simulink model "LoadFlow58BusNetwork_2023"  (R2023b)
settings: Solver=FixedStepDiscrete  StartTime=0.0  StopTime=4.5  FixedStep=75e-6  RelTol=1e-3  EnableMultiTasking=on
undefined symbols (not defined in the file): D1, D11, Delta
libraries: spsSeriesRLCBranchLib x41, spsLoadFlowBusLib x29, spsDistributedParametersLineLib x19, spsThreePhaseSeriesRLCLoadLib x15, spsThreePhaseTransformerTwoWindingsLib x13, spsThreePhaseParallelRLCLoadLib x11, spsThreePhaseVIMeasurementLib x11, spsSynchronousMachinepuStandardLib x7, spsExcitationSystemLib x7, spsHydraulicTurbineandGovernorLib x7, spsGenericPowerSystemStabilizerLib x7, spsMultiBandPowerSystemStabilizerLib x7
(part 2 of 5)

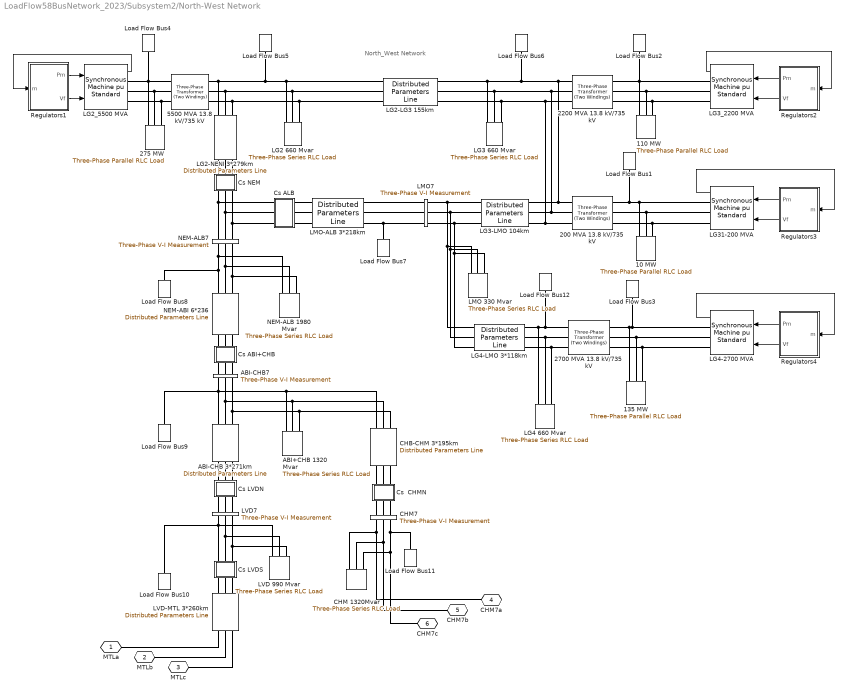
== system LoadFlow58BusNetwork_2023/Subsystem2/North-West Network ==
  note: North_West Network
  10 MW : spsThreePhaseParallelRLCLoadLib/Three-Phase Parallel RLC Load  LConnTagsString=A|B|C  Configuration=Y (grounded)  NominalVoltage=(13800)*1  Vabc=[1e3 1e3 1e3]  Vabcp=[1e3 1e3 1e3]  NominalFrequency=60  UnbalancedPower=off  ActivePower=10000000  InductivePower=0  CapacitivePower=0  Pabc=[10e3 9e3 11e3]  QLabc=[100 90 110]  QCabc=[100 90 110]  Pabcp=[10e3 9e3 11e3]  QLabcp=[100 90 110]  QCabcp=[100 90 110]  Measurements=None  LoadType=constant PQ
  110 MW : spsThreePhaseParallelRLCLoadLib/Three-Phase Parallel RLC Load  LConnTagsString=A|B|C  Configuration=Y (grounded)  NominalVoltage=(13800)*1  Vabc=[1e3 1e3 1e3]  Vabcp=[1e3 1e3 1e3]  NominalFrequency=60  UnbalancedPower=off  ActivePower=110000000  InductivePower=0  CapacitivePower=0  Pabc=[10e3 9e3 11e3]  QLabc=[100 90 110]  QCabc=[100 90 110]  Pabcp=[10e3 9e3 11e3]  QLabcp=[100 90 110]  QCabcp=[100 90 110]  Measurements=None  LoadType=constant PQ
  135 MW : spsThreePhaseParallelRLCLoadLib/Three-Phase Parallel RLC Load  LConnTagsString=A|B|C  Configuration=Y (grounded)  NominalVoltage=(13800)*1  Vabc=[1e3 1e3 1e3]  Vabcp=[1e3 1e3 1e3]  NominalFrequency=60  UnbalancedPower=off  ActivePower=135000000  InductivePower=0  CapacitivePower=0  Pabc=[10e3 9e3 11e3]  QLabc=[100 90 110]  QCabc=[100 90 110]  Pabcp=[10e3 9e3 11e3]  QLabcp=[100 90 110]  QCabcp=[100 90 110]  Measurements=None  LoadType=constant PQ
  200 MVA 13.8 kV/735 kV : spsThreePhaseTransformerTwoWindingsLib/Three-Phase Transformer (Two Windings)  Winding1Connection=Delta (D1)  Winding2Connection=Yg  CoreType=Three single-phase transformers  SetSaturation=off  Hysteresis=off  DataFile='basic_model'  SetInitialFlux=off  Measurements=None  UNITS=pu  NominalPower=[ 200e6 60 ]  Winding1="[ 13.8e3 0.002  0.0]"  Winding2=[ 735e3 0.002 0.12]  Rm=500  Lm=500  L0=0.5  Saturation="[ 0,0  ;  0.005,1.2  ;  1.0,1.4 ]"  InitialFluxes=[ 0.8 , -0.8 , 0.7 ]  BreakLoop=off  DiscreteSolver=Trapezoidal iterative  DataType=off  TransfoNumber=0
  2200 MVA 13.8 kV/735 kV : spsThreePhaseTransformerTwoWindingsLib/Three-Phase Transformer (Two Windings)  Winding1Connection=Delta (D1)  Winding2Connection=Yg  CoreType=Three single-phase transformers  SetSaturation=off  Hysteresis=off  DataFile='basic_model'  SetInitialFlux=off  Measurements=None  UNITS=pu  NominalPower=[ 2200e6 60 ]  Winding1="[ 13.8e3 0.002  0.0]"  Winding2=[ 735e3 0.002 0.12]  Rm=500  Lm=500  L0=0.5  Saturation="[ 0,0  ;  0.005,1.2  ;  1.0,1.4 ]"  InitialFluxes=[ 0.8 , -0.8 , 0.7 ]  BreakLoop=off  DiscreteSolver=Trapezoidal iterative  DataType=off  TransfoNumber=0
  2700 MVA 13.8 kV/735 kV : spsThreePhaseTransformerTwoWindingsLib/Three-Phase Transformer (Two Windings)  Winding1Connection=Delta (D1)  Winding2Connection=Yg  CoreType=Three single-phase transformers  SetSaturation=off  Hysteresis=off  DataFile='basic_model'  SetInitialFlux=off  Measurements=None  UNITS=pu  NominalPower=[ 2700e6 60 ]  Winding1="[ 13.8e3 0.002  0.0]"  Winding2=[ 735e3 0.002 0.12]  Rm=500  Lm=500  L0=0.5  Saturation="[ 0,0  ;  0.005,1.2  ;  1.0,1.4 ]"  InitialFluxes=[ 0.8 , -0.8 , 0.7 ]  BreakLoop=off  DiscreteSolver=Trapezoidal iterative  DataType=off  TransfoNumber=0
  275 MW : spsThreePhaseParallelRLCLoadLib/Three-Phase Parallel RLC Load  LConnTagsString=A|B|C  Configuration=Y (grounded)  NominalVoltage=(13800)*1  Vabc=[1e3 1e3 1e3]  Vabcp=[1e3 1e3 1e3]  NominalFrequency=60  UnbalancedPower=off  ActivePower=275000000  InductivePower=0  CapacitivePower=0  Pabc=[10e3 9e3 11e3]  QLabc=[100 90 110]  QCabc=[100 90 110]  Pabcp=[10e3 9e3 11e3]  QLabcp=[100 90 110]  QCabcp=[100 90 110]  Measurements=None  LoadType=constant PQ
  5500 MVA 13.8 kV/735 kV : spsThreePhaseTransformerTwoWindingsLib/Three-Phase Transformer (Two Windings)  Winding1Connection=Delta (D1)  Winding2Connection=Yg  CoreType=Three single-phase transformers  SetSaturation=off  Hysteresis=off  DataFile='basic_model'  SetInitialFlux=off  Measurements=None  UNITS=pu  NominalPower=[ 5500e6 60 ]  Winding1="[ 13.8e3 0.002  0.0]"  Winding2=[ 735e3 0.002 0.12]  Rm=500  Lm=500  L0=0.5  Saturation="[ 0,0  ;  0.005,1.2  ;  1.0,1.4 ]"  InitialFluxes=[ 0.8 , -0.8 , 0.7 ]  BreakLoop=off  DiscreteSolver=Trapezoidal iterative  DataType=off  TransfoNumber=0
  ABI+CHB 1320 Mvar : spsThreePhaseSeriesRLCLoadLib/Three-Phase Series RLC Load  LConnTagsString=A|B|C  Configuration=Y (grounded)  NominalVoltage=735e3  Vabc=[1e3 1e3 1e3]  Vabcp=[1e3 1e3 1e3]  NominalFrequency=60  UnbalancedPower=off  ActivePower=4400000  InductivePower=1320e6  CapacitivePower=0  Pabc=[10e3 9e3 11e3]  QLabc=[100 90 110]  QCabc=[100 90 110]  Pabcp=[10e3 9e3 11e3]  QLabcp=[100 90 110]  QCabcp=[100 90 110]  Measurements=None  LoadType=constant Z
  ABI-CHB 3*271km : spsDistributedParametersLineLib/Distributed Parameters Line  Phases=3  Length=271  Frequency=60  Resistance="[0.01273  0.3864]/3"  Inductance="[0.9337e-3  4.1264e-3]/3"  Capacitance=[12.74e-9 7.751e-9]*3  x1=[-0.001575 2.66910784944011e-08 -34814.2579740562 -747194.944177999;-0.0015 2.68155154258362e-08 -13676.7298713595 -747880.497252668;-0.001425 2.69185164445309e-08 7471.73119993543 -747968.206100789;-0.00135 2.6999999213047e-08 28614.2194836304 -747458.00060925;-0.001275 2.70598985953061e-08 49733.8339980823 -746350.288628515;-0.0012 2.70981667086584e-08 70813.6920465894 -744645.955646593;-0.001125 2.71147729621596e-08 91836.9427131602 -742346.364081192;-0.00105 2.71097040810249e-08 112786.780332879 -739453.352190625;-0.000975 2.70829641172401e-08 133646.457926094 -735969.232604332;-0.0009 2.70345744463233e-08 154399.300585704 -731896.790474202;-0.000825 2.69645737502369e-08 175028.718806813 -727239.281248164;-0.00075 2.68730179864664e-08 195518.221748137 -722000.428067829;-0.000675 2.67599803432885e-08 215851.430414525 -716184.418792275;-0.0006 2.66255511812656e-08 236012.090750078 -709795.902650327;-0.000525 2.6469837961013e-08 255984.08663139 -702839.986524042;-0.00045 2.62929651572965e-08 275751.452750538 -695322.230866342;-0.000375 2.60950741595291e-08 295298.387377495 -687248.645256074;-0.0003 2.58763231587465e-08 314609.2649918 -678625.683594045;-0.000225 2.56368870211519e-08 333668.648773354 -669460.238943873;-0.00015 2.53769571483301e-08 352461.302942379 -659759.638021774;-7.5e-05 2.50967413242444e-08 370972.204938671 -649531.635339701]  x2=[-0.001575 6.08393924870088e-08 -284619.34107611 -691578.758256664;-0.0015 6.10523834949351e-08 -264954.255311304 -699348.683850969;-0.001425 6.12165701616285e-08 -245077.369168738 -706559.560807798;-0.00135 6.13318212387795e-08 -225004.571927068 -713205.62486244;-0.001275 6.13980445964407e-08 -204751.909473285 -719281.56325298;-0.0012 6.1415187296673e-08 -184335.571475878 -724782.518967232;-0.001125 6.13832356358642e-08 -163771.878443063 -729704.094625366;-0.00105 6.13022151556831e-08 -143077.268676413 -734042.355995104;-0.000975 6.11721906226619e-08 -122268.28513034 -737793.835136684;-0.0009 6.09932659764228e-08 -101361.5621879 -740955.53317508;-0.000825 6.07655842465905e-08 -80373.812363532 -743524.922697255;-0.00075 6.0489327438456e-08 -59321.8129433208 -745499.94977254;-0.000675 6.0164716387485e-08 -38222.3925734968 -746879.035594507;-0.0006 5.97920105827849e-08 -17092.4178078718 -747661.077743053;-0.000525 5.93715079596733e-08 4051.22037502602 -747845.45106565;-0.00045 5.89035446615133e-08 25191.6200743418 -747432.008177083;-0.000375 5.83884947710054e-08 46311.8819780149 -746421.079577273;-0.0003 5.78267700111514e-08 67395.1228718303 -744813.473387074;-0.000225 5.72188194161298e-08 88424.489135602 -742610.474702278;-0.00015 5.65651289723442e-08 109383.170215699 -739813.844566326;-7.5e-05 5.58662212299336e-08 130254.412063144 -736425.81856256]  x3=[-0.001575 1.19957394580366e-10 -354.9640306607 -109.750554354856;-0.0015 1.27832366196785e-10 -351.719210477087 -119.74113183903;-0.001425 1.35605150575568e-10 -348.193231338104 -129.635990094512;-0.00135 1.43269534271808e-10 -344.388911857524 -139.427219323009;-0.001275 1.50819390494449e-10 -340.309293150132 -149.106992565688;-0.0012 1.58248684003943e-10 -335.957636400702 -158.667571959923;-0.001125 1.65551475936731e-10 -331.337420257058 -168.101314924829;-0.00105 1.72721928552677e-10 -326.452338049293 -177.40068027062;-0.000975 1.79754309901672e-10 -321.30629483738 -186.558234226925;-0.0009 1.86642998405664e-10 -315.903404289525 -195.566656385225;-0.000825 1.93382487352465e-10 -310.247985393765 -204.41874555068;-0.00075 1.99967389297728e-10 -304.344559005434 -213.107425498655;-0.000675 2.0639244037159e-10 -298.197844233263 -221.625750631338;-0.0006 2.12652504486529e-10 -291.812754666991 -229.966911529955;-0.000525 2.18742577443073e-10 -285.194394449524 -238.124240398106;-0.00045 2.24657790930084e-10 -278.348054196754 -246.091216391906;-0.000375 2.30393416416404e-10 -271.279206768327 -253.861470832645;-0.0003 2.35944868930779e-10 -263.993502892721 -261.42879229781;-0.000225 2.41307710727008e-10 -256.496766650139 -268.787131586407;-0.00015 2.46477654831413e-10 -248.794990816828 -275.930606554595;-7.5e-05 2.51450568469781e-10 -240.89433207455 -282.853506817784]  x4=[-0.001575 1.87301646960915e-10 -5971.27343085188 -15054.8004559029;-0.0015 1.83445794549808e-10 -5543.27939856518 -15217.5948036273;-0.001425 1.79443298377354e-10 -5110.85415354227 -15368.2244389028;-0.00135 1.75297357977751e-10 -4674.34336990772 -15506.5689507035;-0.001275 1.7101128755232e-10 -4234.09598770311 -15632.5177485434;-0.0012 1.6658851332018e-10 -3790.46393394978 -15745.9701508807;-0.001125 1.62032570779382e-10 -3343.80184132369 -15846.8354656009;-0.00105 1.57347101880685e-10 -2894.46676466753 -15935.0330625145;-0.000975 1.52535852116235e-10 -2442.81789556652 -16010.4924378121;-0.0009 1.4760266752548e-10 -1989.21627521616 -16073.1532704238;-0.000825 1.42551491620702e-10 -1534.02450581142 -16122.9654702385;-0.00075 1.37386362234634e-10 -1077.60646068811 -16159.8892181459;-0.000675 1.32111408292677e-10 -620.326993448042 -16183.894997867;-0.0006 1.26730846512303e-10 -162.551646300739 -16194.9636195487;-0.000525 1.21248978032274e-10 295.353642145493 -16193.0862351041;-0.00045 1.15670184974377e-10 753.022829409257 -16178.2643452858;-0.000375 1.09998926940426e-10 1210.09006174483 -16150.5097984855;-0.0003 1.04239737447318e-10 1666.18996660004 -16109.8447812635;-0.000225 9.83972203030162e-11 2120.95794468951 -16056.3018006122;-0.00015 9.24760459263322e-11 2574.03046144974 -15989.9236579711;-7.5e-05 8.64809476134656e-11 3025.04533764307 -15910.7634150119]  x5=0.00153261764655846  V1=ones(3,3)  V2=ones(3,3)  I1=ones(3,3)  I2=ones(3,3)  nHarmo=1  Measurements=None  Decoupling=on  VsMag0=[610743.955114479 610743.501375024 610743.958218046]  VrMag0=[610622.360478008 610622.247686734 610622.21400369]  VsAngle0=[1.35232982185643 -118.647645266058 121.352379141739]  VrAngle0=[-18.3496130787562 -138.349622838578 101.650391206836]  IsMag0=[305.299965909812 305.301188712511 305.286778309358]  IrMag0=[13308.311716937 13308.3164139131 13308.3246262138]  IsAngle0=[-68.7963830006793 171.200626740014 51.2019231191923]  IrAngle0=[-17.6151010152127 -137.615048514483 102.384907722655]
      settings: AttributesFormatString=\n  LibrarySourceBlock=sps_lib/Power Grid Elements/Distributed Parameters Line
  ABI-CHB7 : spsThreePhaseVIMeasurementLib/Three-Phase V-I Measurement  VoltageMeasurement=no  SetLabelV=on  LabelV=Vabc_ABI7  Vpu=on  VpuLL=off  CurrentMeasurement=no  SetLabelI=off  LabelI=A1  Ipu=off  Pbase=100e6  Vbase=500e3  OutputType=Magnitude  PhasorSimulation=off  PSBequivalent=0
  CHB-CHM 3*195km : spsDistributedParametersLineLib/Distributed Parameters Line  Phases=3  Length=195  Frequency=60  Resistance="[0.01273  0.3864]/3"  Inductance="[0.9337e-3  4.1264e-3]/3"  Capacitance=[12.74e-9 7.751e-9]*3  x1=[-0.001125 2.71147729621596e-08 0 0;-0.00105 2.71097040810249e-08 0 0;-0.000975 2.70829641172401e-08 0 0;-0.0009 2.70345744463233e-08 0 0;-0.000825 2.69645737502369e-08 0 0;-0.00075 2.68730179864664e-08 0 0;-0.000675 2.67599803432885e-08 215851.430414525 -716184.418792275;-0.0006 2.66255511812656e-08 236012.090750078 -709795.902650327;-0.000525 2.6469837961013e-08 255984.08663139 -702839.986524042;-0.00045 2.62929651572965e-08 275751.452750538 -695322.230866342;-0.000375 2.60950741595291e-08 295298.387377495 -687248.645256074;-0.0003 2.58763231587465e-08 314609.2649918 -678625.683594045;-0.000225 2.56368870211519e-08 333668.648773354 -669460.238943873;-0.00015 2.53769571483301e-08 352461.302942379 -659759.638021774;-7.5e-05 2.50967413242444e-08 370972.204938671 -649531.635339701]  x2=[-0.001125 1.81716346267298e-08 0 0;-0.00105 1.81182749100996e-08 0 0;-0.000975 1.80504317217251e-08 0 0;-0.0009 1.79681592944132e-08 0 0;-0.000825 1.78715233954833e-08 0 0;-0.00075 1.77606012741946e-08 0 0;-0.000675 1.76354815999936e-08 127559.107191262 -726636.134488437;-0.0006 1.74962643916335e-08 148050.539525883 -722739.535823106;-0.000525 1.73430609372205e-08 168423.622524456 -718265.190231125;-0.00045 1.7175993705252e-08 188662.07025615 -713216.674435898;-0.000375 1.69951962467171e-08 208749.704415509 -707598.024143708;-0.0003 1.68008130883378e-08 228670.467255135 -701413.730817631;-0.000225 1.65929996170367e-08 248408.434422013 -694668.738087127;-0.00015 1.63719219557232e-08 267947.82768719 -687368.437796186;-7.5e-05 1.61377568304971e-08 287273.027558654 -679518.665693159]  x3=[-0.001125 1.00282083292002e-10 0 0;-0.00105 9.83539884232109e-11 0 0;-0.000975 9.63472708809408e-11 0 0;-0.0009 9.42635348044912e-11 0 0;-0.000825 9.21044459005992e-11 0 0;-0.00075 8.98717301118996e-11 0 0;-0.000675 8.75671722372322e-11 771.180648774941 -4323.83757003434;-0.0006 8.5192614504901e-11 893.110598565729 -4300.30718909173;-0.000525 8.27499551000252e-11 1014.32660940907 -4273.33920837907;-0.00045 8.02411466471593e-11 1134.73178308058 -4242.95518568751;-0.000375 7.76681946493944e-11 1254.22986952666 -4209.17940953991;-0.0003 7.50331558851899e-11 1372.72534380541 -4172.03887977492;-0.000225 7.23381367642166e-11 1490.12348244772 -4131.56328596378;-0.00015 6.95852916435246e-11 1606.33043917781 -4087.78498367688;-7.5e-05 6.67768211053835e-11 1721.25331993251 -4040.73896861923]  x4=[-0.001125 6.8922255092171e-11 0 0;-0.00105 7.14623317195361e-11 0 0;-0.000975 7.39452824523348e-11 0 0;-0.0009 7.6369122457742e-11 0 0;-0.000825 7.87319141551432e-11 0 0;-0.00075 8.10317687650074e-11 0 0;-0.000675 8.32668478187486e-11 979.606952616721 -12037.6056406815;-0.0006 8.54353646283689e-11 1319.52443201704 -12005.1005057404;-0.000525 8.75355857147102e-11 1658.38710377581 -11962.9986771393;-0.00045 8.95658321931705e-11 1995.924086258 -11911.3338104356;-0.000375 9.15244811157788e-11 2331.86555756429 -11850.1472057335;-0.0003 9.34099667685547e-11 2665.9429712226 -11779.4877746684;-0.000225 9.52207819231163e-11 2997.88927086002 -11699.4120013084;-0.00015 9.69554790415353e-11 3327.43910368355 -11609.9838970016;-7.5e-05 9.8612671433477e-11 3654.32903259912 -11511.2749492062]  x5=0.0011028060556417  V1=ones(3,3)  V2=ones(3,3)  I1=ones(3,3)  I2=ones(3,3)  nHarmo=1  Measurements=None  Decoupling=on  VsMag0=[610743.955114479 610743.501375024 610743.958218046]  VrMag0=[602368.350238872 602368.356498677 602368.322152189]  VsAngle0=[1.35232982185643 -118.647645266058 121.352379141739]  VrAngle0=[-5.46332293595376 -125.463326364545 114.536674834105]  IsMag0=[3602.61669203435 3602.60152789052 3602.59275066827]  IrMag0=[9906.44607872208 9906.45414351776 9906.46948058266]  IsAngle0=[-5.30716137481867 -125.307461802351 114.692897272077]  IrAngle0=[-10.7676510977532 -130.767521740257 109.23237318601]
      settings: AttributesFormatString=\n  LibrarySourceBlock=sps_lib/Power Grid Elements/Distributed Parameters Line
  CHM 1320Mvar : spsThreePhaseSeriesRLCLoadLib/Three-Phase Series RLC Load  LConnTagsString=A|B|C  Configuration=Y (grounded)  NominalVoltage=735e3  Vabc=[1e3 1e3 1e3]  Vabcp=[1e3 1e3 1e3]  NominalFrequency=60  UnbalancedPower=off  ActivePower=4400000  InductivePower=1320e6  CapacitivePower=0  Pabc=[10e3 9e3 11e3]  QLabc=[100 90 110]  QCabc=[100 90 110]  Pabcp=[10e3 9e3 11e3]  QLabcp=[100 90 110]  QCabcp=[100 90 110]  Measurements=None  LoadType=constant Z
  CHM7 : spsThreePhaseVIMeasurementLib/Three-Phase V-I Measurement  VoltageMeasurement=no  SetLabelV=on  LabelV=Vabc_CHM7  Vpu=on  VpuLL=off  CurrentMeasurement=no  SetLabelI=off  LabelI=A1  Ipu=off  Pbase=100e6  Vbase=735e3  OutputType=Magnitude  PhasorSimulation=off  PSBequivalent=0
  "Cs  CHMN " : Subsystem  mask{Xc=25/3}
      mask prompts: Xc "Condensator Reactance at  60Hz  (ohm):"
      mask help: Series Compensation
      mask init:
      | Cs=1/Xc/(2*pi*60);
      mask Display: disp('Cs')
  "Cs ABI+CHB " : Subsystem  mask{Xc=25/6}
      mask prompts: Xc "Condensator Reactance at  60Hz  (ohm):"
      mask help: Series Compensation
      mask init:
      | Cs=1/Xc/(2*pi*60);
      mask Display: disp('Cs')
  Cs ALB : Subsystem  mask{Xc=16/3}
      mask prompts: Xc "Reactance @ 60Hz du condensateur (ohm):"
      mask init:
      | Cs=1/Xc/(2*pi*60);
      mask Display: disp('Cs')
  "Cs LVDN " : Subsystem  mask{Xc=34/3}
      mask prompts: Xc "Condensator Reactance at  60Hz  (ohm):"
      mask help: Series Compensation
      mask init:
      | Cs=1/Xc/(2*pi*60);
      mask Display: disp('Cs')
  "Cs LVDS " : Subsystem  mask{Xc=34/3}
      mask prompts: Xc "Condensator Reactance at  60Hz  (ohm):"
      mask help: Series Compensation
      mask init:
      | Cs=1/Xc/(2*pi*60);
      mask Display: disp('Cs')
  "Cs NEM " : Subsystem  mask{Xc=16/3}
      mask prompts: Xc "Condensator Reactance at  60Hz  (ohm):"
      mask help: Series Compensation
      mask init:
      | Cs=1/Xc/(2*pi*60);
      mask Display: disp('Cs')
  LG2 660 Mvar : spsThreePhaseSeriesRLCLoadLib/Three-Phase Series RLC Load  LConnTagsString=A|B|C  Configuration=Y (grounded)  NominalVoltage=735e3  Vabc=[1e3 1e3 1e3]  Vabcp=[1e3 1e3 1e3]  NominalFrequency=60  UnbalancedPower=off  ActivePower=2200000  InductivePower=660e6  CapacitivePower=0  Pabc=[10e3 9e3 11e3]  QLabc=[100 90 110]  QCabc=[100 90 110]  Pabcp=[10e3 9e3 11e3]  QLabcp=[100 90 110]  QCabcp=[100 90 110]  Measurements=None  LoadType=constant Z
  LG2-LG3 155km : spsDistributedParametersLineLib/Distributed Parameters Line  Phases=3  Length=155  Frequency=60  Resistance="[0.01273  0.3864]"  Inductance="[0.9337e-3  4.1264e-3]"  Capacitance=[12.74e-9 7.751e-9]  x1=[-0.0009 5.26292056031291e-10 425726.576739847 -584301.004479606;-0.000825 5.67978956510661e-10 442074.91123427 -572031.87277794;-0.00075 6.09211823302567e-10 458069.857808626 -559305.467549556;-0.000675 6.49957695484177e-10 473698.630347353 -546131.962088074;-0.0006 6.90184001428704e-10 488948.735448812 -532521.887092198;-0.000525 7.29858584842658e-10 503807.982412321 -518486.122247638;-0.00045 7.689497304711e-10 518264.492983209 -504035.887530057;-0.000375 8.07426189450328e-10 532306.71084812 -489182.734235993;-0.0003 8.45257204287745e-10 545923.410872944 -473938.535748927;-0.000225 8.82412533448924e-10 559103.708076024 -458315.478047886;-0.00015 9.18862475532227e-10 571837.066329443 -442326.049966156;-7.5e-05 9.54577893011657e-10 584113.306781438 -425983.033207898]  x2=[-0.0009 -3.11578283864764e-10 428602.512418893 -576982.581433584;-0.000825 -3.58188817976031e-10 444742.80199236 -564635.073573969;-0.00075 -4.04513021426679e-10 460527.570974708 -551836.205075745;-0.000675 -4.50513863357257e-10 475944.201263127 -538596.207158561;-0.0006 -4.96154571398559e-10 490980.369039247 -524925.663674172;-0.000525 -5.41398661066906e-10 505624.054620609 -510835.502645875;-0.00045 -5.86209964929272e-10 519863.552069014 -496336.987532807;-0.000375 -6.30552661514988e-10 533687.478548074 -481441.708226117;-0.0003 -6.74391303950867e-10 547084.783422475 -466161.571784175;-0.000225 -7.17690848296901e-10 560044.757091686 -450508.792914261;-0.00015 -7.60416681559845e-10 572557.03955105 -434495.884208306;-7.5e-05 -8.02534649362315e-10 584611.628673414 -418135.646140526]  x3=[-0.0009 1.07736147592299e-11 1482.81916403309 -2352.94053779552;-0.000825 1.06478201555145e-11 1548.74539245904 -2310.07973089095;-0.00075 1.05135138472838e-11 1613.43357751485 -2265.37228159492;-0.000675 1.03708031969459e-11 1676.83200845517 -2218.85392835833;-0.0006 1.02198022852108e-11 1738.89000554431 -2170.56185724102;-0.000525 1.00606318198972e-11 1799.55796056894 -2120.53467218574;-0.00045 9.89341903943965e-12 1858.78737649404 -2068.81236415879;-0.000375 9.71829761117632e-12 1916.53090623077 -2015.43627918181;-0.0003 9.53540752449756e-12 1972.74239048497 -1960.44908528047;-0.000225 9.34489497894033e-12 2027.37689465619 -1903.89473837623;-0.00015 9.14691226731863e-12 2080.39074475773 -1845.8184471487;-7.5e-05 8.94161765398289e-12 2131.74156232895 -1786.26663689649]  x4=[-0.0009 -1.03438799282861e-11 1223.55408119273 -2231.14873574791;-0.000825 -1.01877994667543e-11 1286.14070278686 -2195.66620561455;-0.00075 -1.00235750342072e-11 1347.69920318179 -2158.42849351123;-0.000675 -9.8513379091437e-12 1408.18037345419 -2119.46536669527;-0.0006 -9.67122577528611e-12 1467.53586588193 -2078.80797169408;-0.000525 -9.48338261151848e-12 1525.71823259253 -2036.48880940715;-0.00045 -9.28795857679182e-12 1582.68096349228 -1992.5417091253;-0.000375 -9.0851098900894e-12 1638.37852344564 -1947.00180148808;-0.0003 -8.87499870554769e-12 1692.76638867538 -1899.90549040089;-0.000225 -8.6577929828328e-12 1745.80108235422 -1851.29042393419;-0.00015 -8.4336663528761e-12 1797.44020935947 -1801.19546422829;-7.5e-05 -8.20279797907634e-12 1847.64249016312 -1749.66065642751]  x5=0.000876589428843401  V1=ones(3,3)  V2=ones(3,3)  I1=ones(3,3)  I2=ones(3,3)  nHarmo=1  Measurements=None  Decoupling=on  VsMag0=[590283.056617351 590282.24389188 590283.87091683]  VrMag0=[586861.315379256 586860.569064556 586862.120536141]  VsAngle0=[25.517390504149 -94.4824726828139 145.517527228789]  VrAngle0=[26.0462334057281 -93.9536337576165 146.046362925441]  IsMag0=[2279.13376434115 2279.13000762777 2279.13554694045]  IrMag0=[2085.26033535305 2085.25824212143 2085.26456016735]  IsAngle0=[21.6590596698404 -98.3408340586402 141.659194593854]  IrAngle0=[18.180207027833 -101.81962572433 138.180340460889]
      settings: AttributesFormatString=\n  LibrarySourceBlock=sps_lib/Power Grid Elements/Distributed Parameters Line
  LG2-NENI 3*279km : spsDistributedParametersLineLib/Distributed Parameters Line  Phases=3  Length=279  Frequency=60  Resistance="[0.01273  0.3864]/3"  Inductance="[0.9337e-3  4.1264e-3]/3"  Capacitance=[12.74e-9 7.751e-9]*3  x1=[-0.00165 9.19274009253425e-11 245808.020606829 -679875.080306766;-0.001575 1.36275318057477e-10 264930.184927492 -672654.157661326;-0.0015 1.80514298785439e-10 283840.568111892 -664895.525574205;-0.001425 2.24608979144913e-10 302524.05348905 -656605.386177183;-0.00135 2.68524110523091e-10 320965.705766622 -647790.366480851;-0.001275 3.12224587835874e-10 339150.782969943 -638457.513077078;-0.0012 3.55675477590337e-10 357064.74822654 -628614.286506079;-0.001125 3.98842045810032e-10 374693.281386679 -618268.555292569;-0.00105 4.41689785800794e-10 392022.290470676 -607428.589655783;-0.000975 4.84184445734868e-10 409037.922933813 -596103.054898396;-0.0009 5.26292056031291e-10 425726.576739847 -584301.004479606;-0.000825 5.67978956510661e-10 442074.91123427 -572031.87277794;-0.00075 6.09211823302567e-10 458069.857808626 -559305.467549556;-0.000675 6.49957695484177e-10 473698.630347353 -546131.962088074;-0.0006 6.90184001428704e-10 488948.735448812 -532521.887092198;-0.000525 7.29858584842658e-10 503807.982412321 -518486.122247638;-0.00045 7.689497304711e-10 518264.492983209 -504035.887530057;-0.000375 8.07426189450328e-10 532306.71084812 -489182.734235993;-0.0003 8.45257204287745e-10 545923.410872944 -473938.535748927;-0.000225 8.82412533448924e-10 559103.708076024 -458315.478047886;-0.00015 9.18862475532227e-10 571837.066329443 -442326.049966156;-7.5e-05 9.54577893011657e-10 584113.306781438 -425983.033207898]  x2=[-0.00165 1.53473828930396e-08 25617.0786734064 -737924.87218899;-0.001575 1.54336529446597e-08 46468.376774716 -736905.697758475;-0.0015 1.55075855702586e-08 67282.528766622 -735297.452188207;-0.001425 1.55691216692267e-08 88042.8961344892 -733101.421085089;-0.00135 1.5618212050548e-08 108732.883358288 -730319.359922783;-0.001275 1.56548174721226e-08 129335.951178799 -726953.492638415;-0.0012 1.56789086721369e-08 149835.629818844 -723006.509854794;-0.001125 1.56904663924539e-08 170215.532148974 -718481.566729565;-0.00105 1.5689481394009e-08 190459.366787089 -713382.28043303;-0.000975 1.56759544641949e-08 210550.951121521 -707712.727256631;-0.0009 1.56498964162322e-08 230474.224247163 -701477.439354431;-0.000825 1.56113280805259e-08 250213.259804316 -694681.401120176;-0.00075 1.55602802880133e-08 269752.278709973 -687330.045202847;-0.000675 1.54967938455187e-08 289075.661771378 -679429.248163885;-0.0006 1.54209195031329e-08 308167.962171768 -670985.325779558;-0.000525 1.53327179136443e-08 327013.917818326 -662005.027992222;-0.00045 1.5232259584054e-08 345598.463542461 -652495.533514525;-0.000375 1.51196248192136e-08 363906.743142674 -642464.444090854;-0.0003 1.49949036576307e-08 381924.121260378 -631919.778420612;-0.000225 1.48581957994936e-08 399636.195079182 -620869.965748197;-0.00015 1.47096105269724e-08 417028.805838279 -609323.839124792;-7.5e-05 1.45492666168606e-08 434088.050150743 -597290.628347358]  x3=[-0.00165 1.12179420312377e-11 -714.300687612479 -1196.52974167796;-0.001575 1.41521917875096e-11 -680.188293409774 -1216.24398928583;-0.0015 1.70751284982023e-11 -645.532167092547 -1234.98599005781;-0.001425 1.99844156124318e-11 -610.36001223792 -1252.74076192527;-0.00135 2.28777274905926e-11 -574.699944928331 -1269.49411199522;-0.001275 2.57527512634383e-11 -538.58047127597 -1285.23264789595;-0.0012 2.86071886809544e-11 -502.030464635428 -1299.94378848267;-0.001125 3.14387579495435e-11 -465.079142522781 -1313.61577389468;-0.00105 3.42451955560569e-11 -427.756043259551 -1326.23767495604;-0.000975 3.70242580772119e-11 -390.091002360226 -1337.79940191216;-0.0009 3.97737239729501e-11 -352.114128682206 -1348.2917124954;-0.000825 4.24913953623027e-11 -313.855780357245 -1357.70621931323;-0.00075 4.51750997803428e-11 -275.346540523621 -1366.03539655295;-0.000675 4.78226919148207e-11 -236.617192878445 -1373.2725859977;-0.0006 5.04320553210936e-11 -197.698697069647 -1379.41200234898;-0.000525 5.30011041139792e-11 -158.622163947303 -1384.44873785129;-0.00045 5.55277846351802e-11 -119.4188306941 -1388.37876621534;-0.000375 5.80100770949473e-11 -80.1200358548099 -1391.19894583659;-0.0003 6.04459971866688e-11 -40.7571942847347 -1392.90702230659;-0.000225 6.28335976730939e-11 -1.36177203715427 -1393.50163021515;-0.00015 6.51709699429255e-11 38.0347387901568 -1392.98229424181;-7.5e-05 6.7456245536534e-11 77.4008452292301 -1391.3494295358]  x4=[-0.00165 4.20570307242303e-11 829.758142042552 -14907.5065102221;-0.001575 4.00130815112291e-11 1250.86903709583 -14878.090885748;-0.0015 3.79371464530884e-11 1670.98000657979 -14836.7819430623;-0.001425 3.5830885020531e-11 2089.75522021334 -14783.6127039016;-0.00135 3.36959809267191e-11 2506.85991549818 -14718.6256709423;-0.001275 3.15341407813202e-11 2921.96066532281 -14641.8727938242;-0.0012 2.93470927262692e-11 3334.72564449908 -14553.4154276228;-0.001125 2.71365850543184e-11 3744.82489501816 -14453.3242838034;-0.00105 2.49043848114789e-11 4151.93058981389 -14341.6793736947;-0.000975 2.26522763844709e-11 4555.7172948228 -14218.5699445298;-0.0009 2.03820600743127e-11 4955.86222913104 -14084.0944081026;-0.000825 1.8095550657187e-11 5352.04552300055 -13938.3602620995;-0.00075 1.57945759337372e-11 5743.95047356801 -13781.4840041669;-0.000675 1.3480975267951e-11 6131.26379801229 -13613.5910387851;-0.0006 1.11565981168015e-11 6513.67588398792 -13434.8155770219;-0.000525 8.82330255181913e-12 6890.88103712448 -13245.300529246;-0.00045 6.48295377377785e-12 7262.57772539398 -13045.1973908869;-0.000375 4.13742262168234e-12 7628.46882015095 -12834.6661213317;-0.0003 1.78858407724775e-12 7988.26183365259 -12613.8750160561;-0.000225 -5.61684233931939e-13 8341.66915286891 -12383.0005720914;-0.00015 -2.91150354332908e-12 8688.40826939625 -12142.2273469357;-7.5e-05 -5.25899544134118e-12 9028.20200529013 -11891.7478110211]  x5=0.00157786097191812  V1=ones(3,3)  V2=ones(3,3)  I1=ones(3,3)  I2=ones(3,3)  nHarmo=1  Measurements=None  Decoupling=on  VsMag0=[590283.056617351 590282.24389188 590283.87091683]  VrMag0=[602875.98020373 602875.441014983 602876.102194664]  VsAngle0=[25.517390504149 -94.4824726828139 145.517527228789]  VrAngle0=[7.62822080532249 -112.371736222197 127.628286669377]  IsMag0=[1145.30812027387 1145.2864371 1145.27794996318]  IrMag0=[12270.9673380092 12270.982090355 12270.9983548867]  IsAngle0=[-25.1951184882343 -145.196235040845 94.8052626724507]  IrAngle0=[8.82574494857738 -111.174127591582 128.82574902524]
      settings: AttributesFormatString=\n  LibrarySourceBlock=sps_lib/Power Grid Elements/Distributed Parameters Line
  LG2_5500 MVA : spsSynchronousMachinepuStandardLib/Synchronous Machine pu Standard  PresetModel=No  MechanicalLoad=Mechanical power Pm  ShowDetailedParameters=on  RotorType=Salient-pole  Units=per unit standard parameters  MeasurementBus=off  NominalParameters="[5500E6  13800   60 ]"  Reactances1=[ 31 32 33 34 35 36 37 ]  Reactances2=[ 1.305, 0.296, 0.252, 0.474, 0.243, 0.18 ]  dAxisTimeConstants=Short-circuit  qAxisTimeConstants=Open-circuit  TimeConstants1=[]  TimeConstants2=[]  TimeConstants3=[]  TimeConstants4=[]  TimeConstants5=[ 1.01, 0.053, 0.1 ]  TimeConstants6=[]  TimeConstants7=[]  TimeConstants8=[]  StatorResistance=2.8544e-3  Mechanical="[ 4.1  0  32]"  PolePairs=32  InitialConditions=[0 -65.2434 0.985682 0.985682 0.985682 -1.22427 -121.224 118.776 1.47412]  SetSaturation=off  Saturation=[0.6404,0.7127,0.8441,0.9214,0.9956,1.082,1.19,1.316,1.457;0.7,0.7698,0.8872,0.9466,0.9969,1.046,1.1,1.151,1.201]  LoadFlowParameters=[2 4000000000 0 0 0]  TsPowergui=0  TsBlock=-1  IterativeModel=Trapezoidal non iterative  IterativeDiscreteModel=Trapezoidal non iterative  BusType=swing  Pref=0  Qref=0  Qmin=-Inf  Qmax=Inf  PLF=0  QLF=0
  LG3 660 Mvar : spsThreePhaseSeriesRLCLoadLib/Three-Phase Series RLC Load  LConnTagsString=A|B|C  Configuration=Y (grounded)  NominalVoltage=735e3  Vabc=[1e3 1e3 1e3]  Vabcp=[1e3 1e3 1e3]  NominalFrequency=60  UnbalancedPower=off  ActivePower=2200000  InductivePower=660e6  CapacitivePower=0  Pabc=[10e3 9e3 11e3]  QLabc=[100 90 110]  QCabc=[100 90 110]  Pabcp=[10e3 9e3 11e3]  QLabcp=[100 90 110]  QCabcp=[100 90 110]  Measurements=None  LoadType=constant Z
  LG3-LMO 104km : spsDistributedParametersLineLib/Distributed Parameters Line  Phases=3  Length=104  Frequency=60  Resistance="[0.01273  0.3864]"  Inductance="[0.9337e-3  4.1264e-3]"  Capacitance=[12.74e-9 7.751e-9]  x1=[-0.0006 -4.96154571398559e-10 0 0;-0.000525 -5.41398661066906e-10 0 0;-0.00045 -5.86209964929272e-10 0 0;-0.000375 -6.30552661514988e-10 533687.478548074 -481441.708226117;-0.0003 -6.74391303950867e-10 547084.783422475 -466161.571784175;-0.000225 -7.17690848296901e-10 560044.757091686 -450508.792914261;-0.00015 -7.60416681559845e-10 572557.03955105 -434495.884208306;-7.5e-05 -8.02534649362315e-10 584611.628673414 -418135.646140526]  x2=[-0.0006 4.38101639813571e-09 0 0;-0.000525 4.31067501405808e-09 0 0;-0.00045 4.23688774232974e-09 0 0;-0.000375 4.15971356736675e-09 480200.396912816 -552194.743514801;-0.0003 4.07921418102375e-09 495619.314773652 -538398.460516428;-0.000225 3.99545393327851e-09 510642.042137488 -524171.790026491;-0.00015 3.90849978079151e-09 525256.570065924 -509526.104627704;-7.5e-05 3.81842123338179e-09 539451.215928944 -494473.111856888]  x3=[-0.0006 1.31198422907821e-11 0 0;-0.000525 1.38206839161878e-11 0 0;-0.00045 1.45104774983345e-11 0 0;-0.000375 1.51886716267867e-11 -139.986222681432 -514.515779236395;-0.0003 1.5854724163535e-11 -125.38405831637 -518.267255559927;-0.000225 1.65081026763724e-11 -110.68166385353 -521.604436969118;-0.00015 1.71482848645127e-11 -95.8907921620919 -524.524655772212;-7.5e-05 1.77747589761098e-11 -81.0232668385779 -527.025577590978]  x4=[-0.0006 -8.37338420658617e-12 0 0;-0.000525 -9.1817004342856e-12 0 0;-0.00045 -9.98267695114259e-12 0 0;-0.000375 -1.07756734687849e-11 3613.50960647485 -3542.5866036648;-0.0003 -1.15600560779296e-11 3712.21557844751 -3439.01470479859;-0.000225 -1.23351977551204e-11 3807.95406208556 -3332.69371019606;-0.00015 -1.31004788639606e-11 3900.64852551002 -3223.70861123352;-7.5e-05 -1.3855287650441e-11 3990.22487018512 -3112.14652893155]  x5=0.000588163229675572  V1=ones(3,3)  V2=ones(3,3)  I1=ones(3,3)  I2=ones(3,3)  nHarmo=1  Measurements=None  Decoupling=on  VsMag0=[586861.315379256 586860.569064556 586862.120536141]  VrMag0=[597501.495499268 597500.918482498 597501.873521823]  VsAngle0=[26.0462334057281 -93.9536337576165 146.046362925441]  VrAngle0=[19.1109154470759 -100.889010750017 139.111000266925]  IsMag0=[436.45107990189 436.445924432075 436.434679859066]  IrMag0=[4141.87607401757 4141.88820061778 4141.89211373212]  IsAngle0=[-37.1184575596894 -157.120552819984 82.8810809575603]  IrAngle0=[23.6678939917987 -96.3319466522304 143.667828394012]
      settings: AttributesFormatString=\n  LibrarySourceBlock=sps_lib/Power Grid Elements/Distributed Parameters Line
  LG31-200 MVA : spsSynchronousMachinepuStandardLib/Synchronous Machine pu Standard  PresetModel=No  MechanicalLoad=Mechanical power Pm  ShowDetailedParameters=on  RotorType=Salient-pole  Units=per unit standard parameters  MeasurementBus=off  NominalParameters="[200E6  13800   60 ]"  Reactances1=[ 31 32 33 34 35 36 37 ]  Reactances2=[ 1.305, 0.296, 0.252, 0.474, 0.243, 0.18 ]  dAxisTimeConstants=Short-circuit  qAxisTimeConstants=Open-circuit  TimeConstants1=[]  TimeConstants2=[]  TimeConstants3=[]  TimeConstants4=[]  TimeConstants5=[ 1.01, 0.053, 0.1 ]  TimeConstants6=[]  TimeConstants7=[]  TimeConstants8=[]  StatorResistance=2.8544e-3  Mechanical="[ 3.2  0  32]"  PolePairs=32  InitialConditions=[0 -67.6291 0.902477 0.902477 0.902477 -4.2812 -124.281 115.719 1.45511]  SetSaturation=off  Saturation=[0.6404,0.7127,0.8441,0.9214,0.9956,1.082,1.19,1.316,1.457;0.7,0.7698,0.8872,0.9466,0.9969,1.046,1.1,1.151,1.201]  LoadFlowParameters=[1 180000000 0 0 0]  TsPowergui=0  TsBlock=-1  IterativeModel=Trapezoidal non iterative  IterativeDiscreteModel=Trapezoidal non iterative  BusType=PV  Pref=180000000  Qref=0  Qmin=-Inf  Qmax=Inf  PLF=0  QLF=0
  LG3_2200 MVA : spsSynchronousMachinepuStandardLib/Synchronous Machine pu Standard  PresetModel=No  MechanicalLoad=Mechanical power Pm  ShowDetailedParameters=on  RotorType=Salient-pole  Units=per unit standard parameters  MeasurementBus=off  NominalParameters="[2200E6  13800   60 ]"  Reactances1=[ 31 32 33 34 35 36 37 ]  Reactances2=[ 1.305, 0.296, 0.252, 0.474, 0.243, 0.18 ]  dAxisTimeConstants=Short-circuit  qAxisTimeConstants=Open-circuit  TimeConstants1=[]  TimeConstants2=[]  TimeConstants3=[]  TimeConstants4=[]  TimeConstants5=[ 1.01, 0.053, 0.1 ]  TimeConstants6=[]  TimeConstants7=[]  TimeConstants8=[]  StatorResistance=2.8544e-3  Mechanical="[ 3.2  0  32]"  PolePairs=32  InitialConditions=[0 -70.0065 0.820496 0.820496 0.820496 -4.90643 -124.906 115.094 1.38903]  SetSaturation=off  Saturation=[0.6404,0.7127,0.8441,0.9214,0.9956,1.082,1.19,1.316,1.457;0.7,0.7698,0.8872,0.9466,0.9969,1.046,1.1,1.151,1.201]  LoadFlowParameters=[1 1800000000 0 0 0]  TsPowergui=0  TsBlock=-1  IterativeModel=Trapezoidal non iterative  IterativeDiscreteModel=Trapezoidal non iterative  BusType=PV  Pref=1800000000  Qref=0  Qmin=-Inf  Qmax=Inf  PLF=0  QLF=0
  LG4 660 Mvar : spsThreePhaseSeriesRLCLoadLib/Three-Phase Series RLC Load  LConnTagsString=A|B|C  Configuration=Y (grounded)  NominalVoltage=735e3  Vabc=[1e3 1e3 1e3]  Vabcp=[1e3 1e3 1e3]  NominalFrequency=60  UnbalancedPower=off  ActivePower=2200000  InductivePower=660e6  CapacitivePower=0  Pabc=[10e3 9e3 11e3]  QLabc=[100 90 110]  QCabc=[100 90 110]  Pabcp=[10e3 9e3 11e3]  QLabcp=[100 90 110]  QCabcp=[100 90 110]  Measurements=None  LoadType=constant Z
  LG4-2700 MVA : spsSynchronousMachinepuStandardLib/Synchronous Machine pu Standard  PresetModel=No  MechanicalLoad=Mechanical power Pm  ShowDetailedParameters=on  RotorType=Salient-pole  Units=per unit standard parameters  MeasurementBus=off  NominalParameters="[2700E6  13800   60 ]"  Reactances1=[ 31 32 33 34 35 36 37 ]  Reactances2=[ 1.305, 0.296, 0.252, 0.474, 0.243, 0.18 ]  dAxisTimeConstants=Short-circuit  qAxisTimeConstants=Open-circuit  TimeConstants1=[]  TimeConstants2=[]  TimeConstants3=[]  TimeConstants4=[]  TimeConstants5=[ 1.01, 0.053, 0.1 ]  TimeConstants6=[]  TimeConstants7=[]  TimeConstants8=[]  StatorResistance=2.8544e-3  Mechanical="[ 3.7  0  32]"  PolePairs=32  InitialConditions=[0 -69.506 0.926038 0.926038 0.926038 -2.40174 -122.402 117.598 1.38766]  SetSaturation=off  Saturation=[0.6404,0.7127,0.8441,0.9214,0.9956,1.082,1.19,1.316,1.457;0.7,0.7698,0.8872,0.9466,0.9969,1.046,1.1,1.151,1.201]  LoadFlowParameters=[1 2500000000 0 0 0]  TsPowergui=0  TsBlock=-1  IterativeModel=Trapezoidal non iterative  IterativeDiscreteModel=Trapezoidal non iterative  BusType=PV  Pref=2500000000  Qref=0  Qmin=-Inf  Qmax=Inf  PLF=0  QLF=0
  LG4-LMO 3*118km : spsDistributedParametersLineLib/Distributed Parameters Line  Phases=3  Length=118  Frequency=60  Resistance="[0.01273  0.3864]/3"  Inductance="[0.9337e-3  4.1264e-3]/3"  Capacitance=[12.74e-9 7.751e-9]*3  x1=[-0.000675 -5.99166742439348e-10 446066.324942456 -570785.422694522;-0.0006 -6.64544644623169e-10 462024.453036378 -557946.706607739;-0.000525 -7.29391319985954e-10 477613.245851754 -544661.976460565;-0.00045 -7.93654931087602e-10 492820.241946124 -530941.851863016;-0.000375 -8.57284106580667e-10 507633.285079485 -516797.300472771;-0.0003 -9.20227982275818e-10 522040.533931802 -502239.629227791;-0.000225 -9.82436241801898e-10 536030.471568783 -487280.475307731;-0.00015 -1.04385915682806e-09 549591.914648333 -471931.796831351;-7.5e-05 -1.10444762681584e-09 562714.022360352 -456205.863297383]  x2=[-0.000675 4.44785566473647e-09 414813.875448599 -602860.773675114;-0.0006 4.38101639813571e-09 431691.280998722 -590892.755025219;-0.000525 4.31067501405808e-09 448223.599143914 -578452.385747919;-0.00045 4.23688774232974e-09 464397.614202001 -565549.610484071;-0.000375 4.15971356736675e-09 480200.396912816 -552194.743514801;-0.0003 4.07921418102375e-09 495619.314773652 -538398.460516428;-0.000225 3.99545393327851e-09 510642.042137488 -524171.790026491;-0.00015 3.90849978079151e-09 525256.570065924 -509526.104627704;-7.5e-05 3.81842123338179e-09 539451.215928944 -494473.111856888]  x3=[-0.000675 1.3268315375682e-11 2040.14143601613 -4504.23210447636;-0.0006 1.513733929628e-11 2166.66257243649 -4444.7556691514;-0.000525 1.69942626594536e-11 2291.45171194749 -4381.72616415155;-0.00045 1.88376010690782e-11 2414.40910002036 -4315.19397429874;-0.000375 2.06658809886331e-11 2535.43644640036 -4245.21228440755;-0.0003 2.24776409191242e-11 2654.43700367859 -4171.83703677014;-0.000225 2.42714325673841e-11 2771.31564463033 -4095.12688643678;-0.00015 2.6045822003815e-11 2885.9789382583 -4015.14315432795;-7.5e-05 2.77993908086504e-11 2998.33522447998 -3931.94977821529]  x4=[-0.000675 -1.60335393599819e-12 6463.18076750054 -9178.78456746785;-0.0006 -4.15089247342358e-12 6720.08725258121 -8992.39755657791;-0.000525 -6.6951128509165e-12 6971.62180273295 -8798.82216066954;-0.00045 -9.23398125763507e-12 7217.58334508497 -8598.21312095242;-0.000375 -1.17654681610209e-11 7457.77526174366 -8390.73080122349;-0.0003 -1.42875499291766e-11 7692.00554696591 -8176.54105967454;-0.000225 -1.67982104485257e-11 7920.08696064553 -7955.81511630776;-0.00015 -1.92954427354635e-11 8141.83717799021 -7728.72941606506;-7.5e-05 -2.17772505407087e-11 8357.0789352691 -7495.46548778069]  x5=0.000667339049054976  V1=ones(3,3)  V2=ones(3,3)  I1=ones(3,3)  I2=ones(3,3)  nHarmo=1  Measurements=None  Decoupling=on  VsMag0=[591479.20702048 591478.775968466 591479.558478766]  VrMag0=[597501.495499268 597500.918482498 597501.873521823]  VsAngle0=[22.5874691411696 -97.4124674392035 142.587537012203]  VrAngle0=[19.1109154470759 -100.889010750017 139.111000266925]  IsMag0=[4048.55267184813 4048.55521766205 4048.56794769896]  IrMag0=[9191.46117506197 9191.4454305139 9191.45421674844]  IsAngle0=[8.9475979222456 -111.052173248445 128.947681135218]  IrAngle0=[19.7310305258233 -100.268962895623 139.731118811244]
      settings: AttributesFormatString=\n  LibrarySourceBlock=sps_lib/Power Grid Elements/Distributed Parameters Line
  LMO 330 Mvar : spsThreePhaseSeriesRLCLoadLib/Three-Phase Series RLC Load  LConnTagsString=A|B|C  Configuration=Y (grounded)  NominalVoltage=735e3  Vabc=[1e3 1e3 1e3]  Vabcp=[1e3 1e3 1e3]  NominalFrequency=60  UnbalancedPower=off  ActivePower=1100000  InductivePower=330e6  CapacitivePower=0  Pabc=[10e3 9e3 11e3]  QLabc=[100 90 110]  QCabc=[100 90 110]  Pabcp=[10e3 9e3 11e3]  QLabcp=[100 90 110]  QCabcp=[100 90 110]  Measurements=None  LoadType=constant Z
  LMO-ALB 3*218km : spsDistributedParametersLineLib/Distributed Parameters Line  Phases=3  Length=218  Frequency=60  Resistance="[0.01273  0.3864]/3"  Inductance="[0.9337e-3  4.1264e-3]/3"  Capacitance=[12.74e-9 7.751e-9]*3  x1=[-0.001275 4.8506885097416e-09 0 0;-0.0012 4.8135461217419e-09 0 0;-0.001125 4.7725558586222e-09 0 0;-0.00105 4.72775048737168e-09 0 0;-0.000975 4.67916582471855e-09 0 0;-0.0009 4.62684070849879e-09 0 0;-0.000825 4.57081696660969e-09 380078.033365271 -625341.876126341;-0.00075 4.51113938357332e-09 397604.874033306 -614346.874646612;-0.000675 4.44785566473647e-09 414813.875448599 -602860.773675114;-0.0006 4.38101639813571e-09 431691.280998722 -590892.755025219;-0.000525 4.31067501405808e-09 448223.599143914 -578452.385747919;-0.00045 4.23688774232974e-09 464397.614202001 -565549.610484071;-0.000375 4.15971356736675e-09 480200.396912816 -552194.743514801;-0.0003 4.07921418102375e-09 495619.314773652 -538398.460516428;-0.000225 3.99545393327851e-09 510642.042137488 -524171.790026491;-0.00015 3.90849978079151e-09 525256.570065924 -509526.104627704;-7.5e-05 3.81842123338179e-09 539451.215928944 -494473.111856888]  x2=[-0.001275 1.60205310998212e-08 0 0;-0.0012 1.60424439969723e-08 0 0;-0.001125 1.60515328098499e-08 0 0;-0.00105 1.60477902729959e-08 0 0;-0.000975 1.60312193781372e-08 0 0;-0.0009 1.60018333717934e-08 0 0;-0.000825 1.59596557446885e-08 256317.712946245 -689303.964750399;-0.00075 1.59047202129722e-08 275702.267037902 -681782.177055774;-0.000675 1.58370706912681e-08 294866.428955675 -673715.383120428;-0.0006 1.57567612575686e-08 313794.879161748 -665110.031416006;-0.000525 1.56638561100064e-08 332472.486542642 -655973.000928995;-0.00045 1.55584295155349e-08 350884.320504794 -646311.595661765;-0.000375 1.54405657505606e-08 369015.662909844 -636133.538793863;-0.0003 1.53103590335739e-08 386852.019840093 -625446.966508217;-0.000225 1.51679134498321e-08 404379.133184716 -614260.421487205;-0.00015 1.50133428681554e-08 421582.99203748 -602582.846083755;-7.5e-05 1.48467708499017e-08 438449.843896845 -590423.575172973]  x3=[-0.001275 2.3839248029739e-11 0 0;-0.0012 2.65658347236236e-11 0 0;-0.001125 2.9271185095701e-11 0 0;-0.00105 3.19531365302771e-11 0 0;-0.000975 3.46095451164103e-11 0 0;-0.0009 3.72382873617211e-11 0 0;-0.000825 3.983726188988e-11 504.220647790102 -2691.25110183847;-0.00075 4.24043911204146e-11 580.102277877382 -2675.92034910895;-0.000675 4.49376229294965e-11 655.520183079589 -2658.4505065953;-0.0006 4.74349322903772e-11 730.414075477238 -2638.85553942234;-0.000525 4.98943228921638e-11 804.72408603866 -2617.15111150701;-0.00045 5.23138287356392e-11 878.390812478394 -2593.35457303689;-0.000375 5.46915157048517e-11 951.355366742463 -2567.48494660074;-0.0003 5.7025483113218e-11 1023.55942208258 -2539.56291198212;-0.000225 5.93138652229028e-11 1094.94525968167 -2509.61078962827;-0.00015 6.15548327362609e-11 1165.4558147934 -2477.65252280753;-7.5e-05 6.37465942581502e-11 1235.03472235885 -2443.71365846941]  x4=[-0.001275 5.75619992930671e-11 0 0;-0.0012 5.53630871459632e-11 0 0;-0.001125 5.31199185940784e-11 0 0;-0.00105 5.08342867920315e-11 0 0;-0.000975 4.85080188389137e-11 0 0;-0.0009 4.61429743177337e-11 0 0;-0.000825 4.37410438088953e-11 4425.6967622701 -12765.9262438956;-0.00075 4.13041473788964e-11 4784.82745779862 -12635.7066271863;-0.000675 3.88342330454576e-11 5140.13323546769 -12495.3862199319;-0.0006 3.63332752203058e-11 5491.330069275 -12345.0771921191;-0.000525 3.38032731308607e-11 5838.1372178451 -12184.899698485;-0.00045 3.12462492220822e-11 6180.27744884975 -12014.9817824671;-0.000375 2.86642475397593e-11 6517.4772606232 -11835.4592738477;-0.0003 2.60593320965307e-11 6849.46710079526 -11646.4756801734;-0.000225 2.34335852219453e-11 7175.98158176731 -11448.1820720374;-0.00015 2.07891058978794e-11 7496.75969285909 -11240.7369623161;-7.5e-05 1.81280080806427e-11 7811.54500895667 -11024.3061794561]  x5=0.00123288061605072  V1=ones(3,3)  V2=ones(3,3)  I1=ones(3,3)  I2=ones(3,3)  nHarmo=1  Measurements=None  Decoupling=on  VsMag0=[597501.495499268 597500.918482498 597501.873521823]  VrMag0=[600465.939453763 600465.308790908 600466.091594142]  VsAngle0=[19.1109154470759 -100.889010750017 139.111000266925]  VrAngle0=[8.21765611493711 -111.782292378914 128.217733982912]  IsMag0=[2247.12525868784 2247.11361991027 2247.12200887511]  IrMag0=[11088.6272022721 11088.6249727987 11088.6349972334]  IsAngle0=[-1.56829194734923 -121.568216294798 118.43200287933]  IrAngle0=[6.94042447158082 -113.05952236936 126.940461027592]
      settings: AttributesFormatString=\n  LibrarySourceBlock=sps_lib/Power Grid Elements/Distributed Parameters Line
  LMO7 : spsThreePhaseVIMeasurementLib/Three-Phase V-I Measurement  VoltageMeasurement=no  SetLabelV=on  LabelV=Vabc_LMO7  Vpu=on  VpuLL=off  CurrentMeasurement=no  SetLabelI=off  LabelI=A1  Ipu=off  Pbase=100e6  Vbase=735e3  OutputType=Magnitude  PhasorSimulation=off  PSBequivalent=0
  LVD 990 Mvar : spsThreePhaseSeriesRLCLoadLib/Three-Phase Series RLC Load  LConnTagsString=A|B|C  Configuration=Y (grounded)  NominalVoltage=735e3  Vabc=[1e3 1e3 1e3]  Vabcp=[1e3 1e3 1e3]  NominalFrequency=60  UnbalancedPower=off  ActivePower=3300000  InductivePower=990e6  CapacitivePower=0  Pabc=[10e3 9e3 11e3]  QLabc=[100 90 110]  QCabc=[100 90 110]  Pabcp=[10e3 9e3 11e3]  QLabcp=[100 90 110]  QCabcp=[100 90 110]  Measurements=None  LoadType=constant Z
  LVD-MTL 3*260km : spsDistributedParametersLineLib/Distributed Parameters Line  Phases=3  Length=260  Frequency=60  Resistance="[0.01273  0.3864]/3"  Inductance="[0.9337e-3  4.1264e-3]/3"  Capacitance=[12.74e-9 7.751e-9]*3  x1=[-0.0015 5.54858366961686e-08 -89258.2599346015 -744297.731345296;-0.001425 5.56883187326623e-08 -68180.8722481362 -746523.607859759;-0.00135 5.5846284379221e-08 -47048.981815598 -748152.724824294;-0.001275 5.59596073605237e-08 -25879.48114687 -749183.779947725;-0.0012 5.60281970879132e-08 -4689.29281688249 -749615.949020362;-0.001125 5.60519987318107e-08 16504.6440620343 -749448.886572861;-0.00105 5.60309932655463e-08 37685.3873810173 -748682.726152386;-0.000975 5.59651974805685e-08 58836.0055779338 -747318.080215854;-0.0009 5.58546639730209e-08 79939.5911722123 -745356.039640348;-0.000825 5.56994811016982e-08 100979.274280424 -742798.172851084;-0.00075 5.54997729174136e-08 121938.236101812 -739646.524567635;-0.000675 5.52556990638337e-08 142799.722362977 -735903.614169419;-0.0006 5.49674546498628e-08 163547.056710994 -731572.433681738;-0.000525 5.4635270093675e-08 184163.65404423 -726656.445384005;-0.00045 5.4259410938522e-08 204633.033770221 -721159.579042049;-0.000375 5.38401776404616e-08 224938.832980007 -715086.228766719;-0.0003 5.33779053281777e-08 245064.819528389 -708441.249501298;-0.000225 5.28729635350838e-08 264994.905009656 -701229.953140541;-0.00015 5.23257559039235e-08 284713.157618418 -693458.104284421;-7.5e-05 5.17367198641044e-08 304203.814885236 -685131.915630001]  x2=[-0.0015 8.54127105066796e-08 -318141.458271983 -654659.491566397;-0.001425 8.56090581434998e-08 -299506.698691673 -663391.865921054;-0.00135 8.57369712091026e-08 -280632.518039035 -671593.934968329;-0.001275 8.57963474517405e-08 -261534.004045298 -679259.142099722;-0.0012 8.57871394069536e-08 -242226.423770331 -686381.359865935;-0.001125 8.57093544355121e-08 -222725.211398391 -692954.894875057;-0.00105 8.55630547175319e-08 -203045.95590027 -698974.492343782;-0.000975 8.53483572027691e-08 -183204.388571708 -704435.340297995;-0.0009 8.50654335171321e-08 -163216.370458044 -709333.073419396;-0.000825 8.47145098254863e-08 -143097.87967513 -713663.776535066;-0.00075 8.42958666508615e-08 -122864.998636675 -717423.987747196;-0.000675 8.38098386502059e-08 -102533.901198207 -720610.701200476;-0.0006 8.3256814346867e-08 -82120.839727942 -723221.369484929;-0.000525 8.26372358200111e-08 -61642.1321148898 -725253.905672274;-0.00045 8.19515983512328e-08 -41114.1487245812 -726706.684984182;-0.000375 8.1200450028634e-08 -20553.2993128498 -727578.546091098;-0.0003 8.03843913086909e-08 23.9800918763358 -727868.792040595;-0.000225 7.95040745362581e-08 20601.2403272839 -727577.1908145;-0.00015 7.85602034230941e-08 41162.0322463834 -726703.975514372;-7.5e-05 7.75535324853251e-08 61689.9198667053 -725249.844175161]  x3=[-0.0015 2.42299174427483e-10 326.034617914414 -307.945403569631;-0.001425 2.50521046839075e-10 334.610417599465 -298.60457274333;-0.00135 2.58542656558925e-10 342.918734836399 -289.025041990382;-0.001275 2.66357591234957e-10 350.952928083537 -279.214469041097;-0.0012 2.73959603727964e-10 358.706574929725 -269.180696317386;-0.001125 2.81342617105473e-10 366.173477228308 -258.931744663641;-0.00105 2.88500729499554e-10 373.347666051838 -248.475806935001;-0.000975 2.95428218824682e-10 380.223406463536 -237.821241448104;-0.0009 3.02119547351885e-10 386.795202101721 -226.976565299581;-0.000825 3.0856936613552e-10 393.05779957351 -215.950447557615;-0.00075 3.14772519289135e-10 399.006192654307 -204.751702332024;-0.000675 3.20724048107011e-10 404.635626289695 -193.389281728395;-0.0006 3.26419195028073e-10 409.94160039656 -181.872268691908;-0.000525 3.31853407439011e-10 414.919873460385 -170.209869746567;-0.00045 3.3702234131357e-10 419.566465925852 -158.41140763565;-0.000375 3.41921864685097e-10 423.877663378041 -146.486313869244;-0.0003 3.46548060949575e-10 427.85001951167 -134.444121184846;-0.000225 3.50897231996493e-10 431.480358886027 -122.294455927038;-0.00015 3.54965901165061e-10 434.765779463362 -110.04703035233;-7.5e-05 3.58750816023397e-10 437.703654928732 -97.7116348653337]  x4=[-0.0015 2.62842048137477e-10 -7428.61939570767 -14286.168118043;-0.001425 2.60300013001731e-10 -7021.77252832244 -14490.4696992902;-0.00135 2.57549898018315e-10 -6609.31256341479 -14683.1878207715;-0.001275 2.54593901587069e-10 -6191.56921516982 -14864.1684265692;-0.0012 2.51434386686312e-10 -5768.87642122843 -15033.266843556;-0.001125 2.48073878983913e-10 -5341.57207574268 -15190.3478970449;-0.00105 2.44515064818311e-10 -4909.99775926837 -15335.2860188449;-0.000975 2.407607890511e-10 -4474.49846571079 -15467.9653476392;-0.0009 2.36814052792885e-10 -4035.42232654184 -15588.2798216025;-0.000825 2.32678011004244e-10 -3593.12033250909 -15696.133263185;-0.00075 2.28355969973699e-10 -3147.94605305911 -15791.4394559958;-0.000675 2.23851384674721e-10 -2700.2553536995 -15874.1222137226;-0.0006 2.19167856003874e-10 -2250.40611152545 -15944.115441034;-0.000525 2.14309127902319e-10 -1798.7579291382 -16001.363186415;-0.00045 2.09279084362958e-10 -1345.67184718433 -16045.8196868938;-0.000375 2.04081746325635e-10 -891.51005574528 -16077.4494046242;-0.0003 1.98721268462855e-10 -436.635604808232 -16096.2270552937;-0.000225 1.93201935858603e-10 18.587885950551 -16102.1376283358;-0.00015 1.87528160582914e-10 473.79651783771 -16095.1763989288;-7.5e-05 1.81704478164932e-10 928.626404037838 -16075.3489317729]  x5=0.00147040807418893  V1=ones(3,3)  V2=ones(3,3)  I1=ones(3,3)  I2=ones(3,3)  nHarmo=1  Measurements=None  Decoupling=on  VsMag0=[612070.919184167 612070.52687088 612070.83212123]  VrMag0=[594302.51828104 594302.525591461 594302.38038744]  VsAngle0=[-4.43840982431777 -124.438398032267 115.561627875914]  VrAngle0=[-23.5181046800016 -143.518120437638 96.4818868308225]  IsMag0=[368.438417397958 368.422778585345 368.434712933272]  IrMag0=[13227.952080821 13227.9561692164 13227.9649229577]  IsAngle0=[49.0336389583768 -70.965622160566 169.036114575874]  IrAngle0=[-25.0738913250263 -145.07383731925 94.9261203418314]
      settings: AttributesFormatString=\n  LibrarySourceBlock=sps_lib/Power Grid Elements/Distributed Parameters Line
  LVD7 : spsThreePhaseVIMeasurementLib/Three-Phase V-I Measurement  VoltageMeasurement=no  SetLabelV=on  LabelV=Vabc_LVD7  Vpu=on  VpuLL=off  CurrentMeasurement=no  SetLabelI=off  LabelI=A1  Ipu=off  Pbase=100e6  Vbase=735e3  OutputType=Magnitude  PhasorSimulation=off  PSBequivalent=0
  Load Flow Bus1 : spsLoadFlowBusLib/Load Flow Bus  LConnTagsString=a  Phases=single  Connectors=on one side  ID=LG31_13.8  Vbase=13.8e3  Vref=1  Vangle=0  VLF=1  VLFb=1  VLFc=1  angleLF=-0.0351  angleLFb=0  angleLFc=0
      settings: AttributesFormatString=%<ID>\n%<Vbase>V\n%<VLF>pu\n%<angleLF>deg.
  Load Flow Bus10 : spsLoadFlowBusLib/Load Flow Bus  LConnTagsString=a  Phases=single  Connectors=on one side  ID=LVD7  Vbase=735e3  Vref=1  Vangle=0  VLF=1.05  VLFb=1  VLFc=1  angleLF=-12.02  angleLFb=0  angleLFc=0
      settings: AttributesFormatString=%<ID>\n%<Vbase>V\n%<VLF>pu\n%<angleLF>deg.
  Load Flow Bus11 : spsLoadFlowBusLib/Load Flow Bus  LConnTagsString=a  Phases=single  Connectors=on one side  ID=CHM7  Vbase=735e3  Vref=1  Vangle=0  VLF=1.047  VLFb=1  VLFc=1  angleLF=-4.064  angleLFb=0  angleLFc=0
      settings: AttributesFormatString=%<ID>\n%<Vbase>V\n%<VLF>pu\n%<angleLF>deg.
  Load Flow Bus12 : spsLoadFlowBusLib/Load Flow Bus  LConnTagsString=a  Phases=single  Connectors=on one side  ID=LG47  Vbase=735e3  Vref=1  Vangle=0  VLF=1.004  VLFb=1  VLFc=1  angleLF=20.71  angleLFb=0  angleLFc=0
      settings: AttributesFormatString=%<ID>\n%<Vbase>V\n%<VLF>pu\n%<angleLF>deg.
  Load Flow Bus2 : spsLoadFlowBusLib/Load Flow Bus  LConnTagsString=a  Phases=single  Connectors=on one side  ID=LG3_13.8  Vbase=13.8e3  Vref=1  Vangle=0  VLF=1  VLFb=1  VLFc=1  angleLF=-0.6025  angleLFb=0  angleLFc=0
      settings: AttributesFormatString=%<ID>\n%<Vbase>V\n%<VLF>pu\n%<angleLF>deg.
  Load Flow Bus3 : spsLoadFlowBusLib/Load Flow Bus  LConnTagsString=a  Phases=single  Connectors=on one side  ID=LG4_13.8  Vbase=13.8e3  Vref=1  Vangle=0  VLF=1  VLFb=1  VLFc=1  angleLF=-3.293  angleLFb=0  angleLFc=0
      settings: AttributesFormatString=%<ID>\n%<Vbase>V\n%<VLF>pu\n%<angleLF>deg.
  Load Flow Bus4 : spsLoadFlowBusLib/Load Flow Bus  LConnTagsString=a  Phases=single  Connectors=on one side  ID=LG2_13.8  Vbase=13.8e3  Vref=1  Vangle=0  VLF=1  VLFb=1  VLFc=1  angleLF=0  angleLFb=0  angleLFc=0
      settings: AttributesFormatString=%<ID>\n%<Vbase>V\n%<VLF>pu\n%<angleLF>deg.
  Load Flow Bus5 : spsLoadFlowBusLib/Load Flow Bus  LConnTagsString=a  Phases=single  Connectors=on one side  ID=LG27  Vbase=735e3  Vref=1  Vangle=0  VLF=1  VLFb=1  VLFc=1  angleLF=23.57  angleLFb=0  angleLFc=0
      settings: AttributesFormatString=%<ID>\n%<Vbase>V\n%<VLF>pu\n%<angleLF>deg.
  Load Flow Bus6 : spsLoadFlowBusLib/Load Flow Bus  LConnTagsString=a  Phases=single  Connectors=on one side  ID=LG37  Vbase=735e3  Vref=1  Vangle=0  VLF=0.994  VLFb=1  VLFc=1  angleLF=24.1  angleLFb=0  angleLFc=0
      settings: AttributesFormatString=%<ID>\n%<Vbase>V\n%<VLF>pu\n%<angleLF>deg.
  Load Flow Bus7 : spsLoadFlowBusLib/Load Flow Bus  LConnTagsString=a  Phases=single  Connectors=on one side  ID=LMO7  Vbase=735e3  Vref=1  Vangle=0  VLF=1.016  VLFb=1  VLFc=1  angleLF=17.31  angleLFb=0  angleLFc=0
      settings: AttributesFormatString=%<ID>\n%<Vbase>V\n%<VLF>pu\n%<angleLF>deg.
  Load Flow Bus8 : spsLoadFlowBusLib/Load Flow Bus  LConnTagsString=a  Phases=single  Connectors=on one side  ID=NEM_ALB7  Vbase=735e3  Vref=1  Vangle=0  VLF=1.028  VLFb=1  VLFc=1  angleLF=8.928  angleLFb=0  angleLFc=0
      settings: AttributesFormatString=%<ID>\n%<Vbase>V\n%<VLF>pu\n%<angleLF>deg.
  Load Flow Bus9 : spsLoadFlowBusLib/Load Flow Bus  LConnTagsString=a  Phases=single  Connectors=on one side  ID=ABI_CHB7  Vbase=735e3  Vref=1  Vangle=0  VLF=1.046  VLFb=1  VLFc=1  angleLF=0.1334  angleLFb=0  angleLFc=0
      settings: AttributesFormatString=%<ID>\n%<Vbase>V\n%<VLF>pu\n%<angleLF>deg.
  NEM-ABI 6*236 : spsDistributedParametersLineLib/Distributed Parameters Line  Phases=3  Length=236  Frequency=60  Resistance="[0.01273  0.3864]/6"  Inductance="[0.9337e-3  4.1264e-3]/6"  Capacitance=[12.74e-9 7.751e-9]*6  x1=[-0.00135 1.54480419099584e-08 0 0;-0.001275 1.54933374005031e-08 0 0;-0.0012 1.5526247754186e-08 0 0;-0.001125 1.55467466629737e-08 0 0;-0.00105 1.55548177403522e-08 0 0;-0.000975 1.55504545344257e-08 0 0;-0.0009 1.55336605330744e-08 0 0;-0.000825 1.55044491611659e-08 284117.477880586 -680689.106292079;-0.00075 1.5462843769824e-08 303247.373018727 -672384.845537111;-0.000675 1.5408877617762e-08 322134.856846718 -663543.090624454;-0.0006 1.5342593844696e-08 340764.830998974 -654170.909517701;-0.000525 1.52640454368602e-08 359122.402959206 -644275.794195031;-0.00045 1.51732951846498e-08 377192.897965269 -633865.654660231;-0.000375 1.50704156324281e-08 394961.870739944 -622948.812619565;-0.0003 1.49554890205349e-08 412415.117038268 -611533.994829528;-0.000225 1.48286072195453e-08 429538.685002195 -599630.326120808;-0.00015 1.46898716568297e-08 446318.886313494 -587247.322104039;-7.5e-05 1.45393932354742e-08 462742.307135981 -574394.881563165]  x2=[-0.00135 2.80886171220477e-08 0 0;-0.001275 2.81435828057667e-08 0 0;-0.0012 2.81760509400021e-08 0 0;-0.001125 2.81859955702241e-08 0 0;-0.00105 2.81734087468474e-08 0 0;-0.000975 2.81383005315861e-08 0 0;-0.0009 2.80806989894103e-08 0 0;-0.000825 2.80006501661115e-08 125357.104454011 -735061.346284943;-0.00075 2.78982180514942e-08 146087.597415356 -731223.617196998;-0.000675 2.77734845282236e-08 166701.310186542 -726801.359137561;-0.0006 2.76265493063697e-08 187181.764480981 -721798.107192065;-0.000525 2.74575298437006e-08 207512.588536871 -716217.86088356;-0.00045 2.72665612517888e-08 227677.530204534 -710065.080975565;-0.000375 2.70537961880047e-08 247660.469938134 -703344.685906199;-0.0003 2.68194047334848e-08 267445.433681397 -696062.047856453;-0.000225 2.65635742571717e-08 287016.605637029 -688222.988455758;-0.00015 2.62865092660337e-08 306358.340909615 -679833.774128256;-7.5e-05 2.59884312415855e-08 325455.178011918 -670901.111083522]  x3=[-0.00135 1.4521579015846e-10 0 0;-0.001275 1.51977599316037e-10 0 0;-0.0012 1.58617919906056e-10 0 0;-0.001125 1.65131443757838e-10 0 0;-0.00105 1.71512964060075e-10 0 0;-0.000975 1.7775737952308e-10 0 0;-0.0009 1.83859698456672e-10 0 0;-0.000825 1.89815042760466e-10 -448.187482109773 -4499.57322109661;-0.00075 1.95618651823345e-10 -320.801895602807 -4510.44404859877;-0.000675 2.01265886329022e-10 -193.159864968931 -4517.7092961406;-0.0006 2.06752231964639e-10 -65.363425294443 -4521.36315599436;-0.000525 2.12073303029439e-10 62.4852649021311 -4521.40270732039;-0.00045 2.17224845940627e-10 190.284005333999 -4517.82791850198;-0.000375 2.22202742633622e-10 317.930635643446 -4510.64164717059;-0.0003 2.27003013853972e-10 445.323117067262 -4499.8496379216;-0.000225 2.31621822338309e-10 572.359614004966 -4485.46051772205;-0.00015 2.36055475881802e-10 698.93857542463 -4467.48578901449;-7.5e-05 2.40300430289644e-10 824.958816041218 -4445.93982052201]  x4=[-0.00135 1.64946608320876e-10 0 0;-0.001275 1.61480469500831e-10 0 0;-0.0012 1.57885245664201e-10 0 0;-0.001125 1.54163810777912e-10 0 0;-0.00105 1.50319139700072e-10 0 0;-0.000975 1.46354305801916e-10 0 0;-0.0009 1.42272478510998e-10 0 0;-0.000825 1.38076920777601e-10 4622.2243852515 -28011.6084746955;-0.00075 1.33770986466381e-10 5412.27949589223 -27869.7398149546;-0.000675 1.29358117675345e-10 6198.0081131146 -27705.592511627;-0.0006 1.24841841984285e-10 6978.78213748405 -27519.2977815554;-0.000525 1.20225769634887e-10 7753.97743019174 -27311.0045458966;-0.00045 1.15513590644759e-10 8522.97431198156 -27080.8793110762;-0.000375 1.10709071857686e-10 9285.15805851227 -26829.1060356858;-0.0003 1.05816053932476e-10 10039.9193917587 -26555.8859834296;-0.000225 1.00838448272793e-10 10786.6549670593 -26261.437562237;-0.00015 9.57802339004398e-11 11524.7678554205 -25945.9961496706;-7.5e-05 9.06454542745936e-11 12253.668020693 -25609.8139047691]  x5=0.00133467809810995  V1=ones(3,3)  V2=ones(3,3)  I1=ones(3,3)  I2=ones(3,3)  nHarmo=1  Measurements=None  Decoupling=on  VsMag0=[602251.717194387 602251.086049828 602251.913986818]  VrMag0=[608840.309919311 608839.972623148 608840.270927367]  VsAngle0=[10.4755045319366 -109.524439182992 130.475584674525]  VrAngle0=[-2.50190241955067 -122.50188833051 117.498132114116]  IsMag0=[3712.6438895587 3712.61521802382 3712.60597455424]  IrMag0=[23309.6118788337 23309.6245706253 23309.6488489225]  IsAngle0=[-17.8678983044397 -137.868318490081 102.132274803411]  IrAngle0=[-2.81003503241439 -122.809948112048 117.189981410573]
      settings: AttributesFormatString=\n  LibrarySourceBlock=sps_lib/Power Grid Elements/Distributed Parameters Line
  NEM-ALB 1980 Mvar : spsThreePhaseSeriesRLCLoadLib/Three-Phase Series RLC Load  LConnTagsString=A|B|C  Configuration=Y (grounded)  NominalVoltage=735e3  Vabc=[1e3 1e3 1e3]  Vabcp=[1e3 1e3 1e3]  NominalFrequency=60  UnbalancedPower=off  ActivePower=6600000  InductivePower=1980e6  CapacitivePower=0  Pabc=[10e3 9e3 11e3]  QLabc=[100 90 110]  QCabc=[100 90 110]  Pabcp=[10e3 9e3 11e3]  QLabcp=[100 90 110]  QCabcp=[100 90 110]  Measurements=None  LoadType=constant Z
  NEM-ALB7 : spsThreePhaseVIMeasurementLib/Three-Phase V-I Measurement  VoltageMeasurement=no  SetLabelV=on  LabelV=Vabc_NEM7  Vpu=on  VpuLL=off  CurrentMeasurement=no  SetLabelI=off  LabelI=A1  Ipu=off  Pbase=100e6  Vbase=735e3  OutputType=Magnitude  PhasorSimulation=off  PSBequivalent=0
  Regulators1 : Subsystem
  Regulators2 : Subsystem
  Regulators3 : Subsystem
  Regulators4 : Subsystem
  MTLa : PMIOPort  Side=Right
  MTLb : PMIOPort  Port=2  Side=Right
  MTLc : PMIOPort  Port=3  Side=Right
  CHM7a : PMIOPort  Port=4  Side=Right
  CHM7b : PMIOPort  Port=5  Side=Right
  CHM7c : PMIOPort  Port=6  Side=Right
  wires:
  Regulators2/1(Pm) -> LG3_2200 MVA/1
  Regulators4/2(Vf) -> LG4-2700 MVA/2
  Regulators4/1(Pm) -> LG4-2700 MVA/1
  Regulators3/2(Vf) -> LG31-200 MVA/2
  Regulators3/1(Pm) -> LG31-200 MVA/1
  Regulators2/2(Vf) -> LG3_2200 MVA/2
  LG3_2200 MVA/1 -> Regulators2/1(m)
  Regulators1/1(Pm) -> LG2_5500 MVA/1
  Regulators1/2(Vf) -> LG2_5500 MVA/2
  LG2_5500 MVA/1 -> Regulators1/1(m)
  LG31-200 MVA/1 -> Regulators3/1(m)
  LG4-2700 MVA/1 -> Regulators4/1(m)
  connections:
  LG2-NENI 3*279km/RConn1 -- "Cs NEM "/LConn1
  LG2-NENI 3*279km/RConn2 -- "Cs NEM "/LConn2
  LG2-NENI 3*279km/RConn3 -- "Cs NEM "/LConn3
  CHB-CHM 3*195km/RConn1 -- "Cs  CHMN "/LConn1
  CHB-CHM 3*195km/RConn2 -- "Cs  CHMN "/LConn2
  CHB-CHM 3*195km/RConn3 -- "Cs  CHMN "/LConn3
  Load Flow Bus2/LConn1 -- 2200 MVA 13.8 kV/735 kV/LConn1 -- LG3_2200 MVA/RConn1 -- 110 MW/LConn1
  2200 MVA 13.8 kV/735 kV/LConn2 -- LG3_2200 MVA/RConn2 -- 110 MW/LConn2
  2200 MVA 13.8 kV/735 kV/LConn3 -- LG3_2200 MVA/RConn3 -- 110 MW/LConn3
  Load Flow Bus1/LConn1 -- 200 MVA 13.8 kV/735 kV/LConn1 -- LG31-200 MVA/RConn1 -- 10 MW/LConn1
  200 MVA 13.8 kV/735 kV/LConn2 -- LG31-200 MVA/RConn2 -- 10 MW/LConn2
  200 MVA 13.8 kV/735 kV/LConn3 -- LG31-200 MVA/RConn3 -- 10 MW/LConn3
  Load Flow Bus6/LConn1 -- 2200 MVA 13.8 kV/735 kV/RConn1 -- 200 MVA 13.8 kV/735 kV/RConn1 -- LG3-LMO 104km/LConn1 -- LG3 660 Mvar/LConn1 -- LG2-LG3 155km/RConn1
  2200 MVA 13.8 kV/735 kV/RConn2 -- LG3 660 Mvar/LConn2 -- LG2-LG3 155km/RConn2 -- 200 MVA 13.8 kV/735 kV/RConn2 -- LG3-LMO 104km/LConn2
  LG3-LMO 104km/RConn1 -- LMO7/RConn1 -- LG4-LMO 3*118km/RConn1 -- LMO 330 Mvar/LConn1
  LG3-LMO 104km/RConn2 -- LMO7/RConn2 -- LG4-LMO 3*118km/RConn2 -- LMO 330 Mvar/LConn2
  LG3-LMO 104km/RConn3 -- LMO7/RConn3 -- LG4-LMO 3*118km/RConn3 -- LMO 330 Mvar/LConn3
  LG4-LMO 3*118km/LConn1 -- LG4 660 Mvar/LConn1 -- 2700 MVA 13.8 kV/735 kV/RConn1 -- Load Flow Bus12/LConn1
  LG4-LMO 3*118km/LConn2 -- 2700 MVA 13.8 kV/735 kV/RConn2 -- LG4 660 Mvar/LConn2
  LG4 660 Mvar/LConn3 -- 2700 MVA 13.8 kV/735 kV/RConn3 -- LG4-LMO 3*118km/LConn3
  Load Flow Bus3/LConn1 -- LG4-2700 MVA/RConn1 -- 2700 MVA 13.8 kV/735 kV/LConn1 -- 135 MW/LConn1
  LG4-2700 MVA/RConn2 -- 2700 MVA 13.8 kV/735 kV/LConn2 -- 135 MW/LConn2
  LG4-2700 MVA/RConn3 -- 2700 MVA 13.8 kV/735 kV/LConn3 -- 135 MW/LConn3
  Load Flow Bus4/LConn1 -- 5500 MVA 13.8 kV/735 kV/LConn1 -- LG2_5500 MVA/RConn1 -- 275 MW/LConn1
  5500 MVA 13.8 kV/735 kV/LConn2 -- LG2_5500 MVA/RConn2 -- 275 MW/LConn2
  LG2_5500 MVA/RConn3 -- 5500 MVA 13.8 kV/735 kV/LConn3 -- 275 MW/LConn3
  5500 MVA 13.8 kV/735 kV/RConn1 -- LG2-NENI 3*279km/LConn1 -- LG2-LG3 155km/LConn1 -- LG2 660 Mvar/LConn1 -- Load Flow Bus5/LConn1
  LG2-LG3 155km/LConn2 -- 5500 MVA 13.8 kV/735 kV/RConn2 -- LG2-NENI 3*279km/LConn2 -- LG2 660 Mvar/LConn2
  LG2-LG3 155km/LConn3 -- 5500 MVA 13.8 kV/735 kV/RConn3 -- LG2-NENI 3*279km/LConn3 -- LG2 660 Mvar/LConn3
  "Cs NEM "/RConn1 -- NEM-ALB7/LConn1 -- Cs ALB/RConn1
  "Cs NEM "/RConn2 -- NEM-ALB7/LConn2 -- Cs ALB/RConn2
  "Cs NEM "/RConn3 -- NEM-ALB7/LConn3 -- Cs ALB/RConn3
  LMO7/LConn1 -- LMO-ALB 3*218km/LConn1
  LMO7/LConn2 -- LMO-ALB 3*218km/LConn2
  Load Flow Bus7/LConn1 -- LMO7/LConn3 -- LMO-ALB 3*218km/LConn3
  Cs ALB/LConn1 -- LMO-ALB 3*218km/RConn1
  Cs ALB/LConn2 -- LMO-ALB 3*218km/RConn2
  Cs ALB/LConn3 -- LMO-ALB 3*218km/RConn3
  200 MVA 13.8 kV/735 kV/RConn3 -- LG3-LMO 104km/LConn3 -- LG3 660 Mvar/LConn3 -- LG2-LG3 155km/RConn3 -- 2200 MVA 13.8 kV/735 kV/RConn3
  Load Flow Bus8/LConn1 -- NEM-ABI 6*236/LConn1 -- NEM-ALB7/RConn1 -- NEM-ALB 1980 Mvar/LConn1
  NEM-ALB 1980 Mvar/LConn2 -- NEM-ALB7/RConn2 -- NEM-ABI 6*236/LConn2
  NEM-ALB 1980 Mvar/LConn3 -- NEM-ALB7/RConn3 -- NEM-ABI 6*236/LConn3
  NEM-ABI 6*236/RConn1 -- "Cs ABI+CHB "/LConn1
  NEM-ABI 6*236/RConn2 -- "Cs ABI+CHB "/LConn2
  NEM-ABI 6*236/RConn3 -- "Cs ABI+CHB "/LConn3
  "Cs ABI+CHB "/RConn1 -- ABI-CHB7/LConn1
  "Cs ABI+CHB "/RConn2 -- ABI-CHB7/LConn2
  "Cs ABI+CHB "/RConn3 -- ABI-CHB7/LConn3
  Load Flow Bus9/LConn1 -- ABI+CHB 1320 Mvar/LConn1 -- CHB-CHM 3*195km/LConn1 -- ABI-CHB 3*271km/LConn1 -- ABI-CHB7/RConn1
  ABI-CHB 3*271km/LConn2 -- ABI-CHB7/RConn2 -- ABI+CHB 1320 Mvar/LConn2 -- CHB-CHM 3*195km/LConn2
  ABI-CHB 3*271km/LConn3 -- ABI-CHB7/RConn3 -- ABI+CHB 1320 Mvar/LConn3 -- CHB-CHM 3*195km/LConn3
  ABI-CHB 3*271km/RConn1 -- "Cs LVDN "/LConn1
  ABI-CHB 3*271km/RConn2 -- "Cs LVDN "/LConn2
  ABI-CHB 3*271km/RConn3 -- "Cs LVDN "/LConn3
  "Cs LVDN "/RConn1 -- LVD7/LConn1
  "Cs LVDN "/RConn2 -- LVD7/LConn2
  "Cs LVDN "/RConn3 -- LVD7/LConn3
  "Cs LVDS "/LConn1 -- LVD 990 Mvar/LConn1 -- Load Flow Bus10/LConn1 -- LVD7/RConn1
  "Cs LVDS "/LConn2 -- LVD7/RConn2 -- LVD 990 Mvar/LConn2
  "Cs LVDS "/LConn3 -- LVD7/RConn3 -- LVD 990 Mvar/LConn3
  "Cs LVDS "/RConn1 -- LVD-MTL 3*260km/LConn1
  "Cs LVDS "/RConn2 -- LVD-MTL 3*260km/LConn2
  "Cs LVDS "/RConn3 -- LVD-MTL 3*260km/LConn3
  MTLa/RConn1 -- LVD-MTL 3*260km/RConn1
  MTLb/RConn1 -- LVD-MTL 3*260km/RConn2
  MTLc/RConn1 -- LVD-MTL 3*260km/RConn3
  "Cs  CHMN "/RConn1 -- CHM7/LConn1
  "Cs  CHMN "/RConn2 -- CHM7/LConn2
  "Cs  CHMN "/RConn3 -- CHM7/LConn3
  CHM 1320Mvar/LConn2 -- CHM7/RConn2 -- CHM7b/RConn1
  Load Flow Bus11/LConn1 -- CHM 1320Mvar/LConn3 -- CHM7c/RConn1 -- CHM7/RConn3
  CHM7a/RConn1 -- CHM 1320Mvar/LConn1 -- CHM7/RConn1
